simulink model "Tutorial3_part2"  (R2020b)
settings: Solver=FixedStepAuto  StartTime=0.0  StopTime=inf  RelTol=1e-3  EnableMultiTasking=on
settings Model: SILPILModeSetting=veronly  EnablePacing=on  ExtModeTrigDuration=2  Creator=helve  LastModifiedBy=helve
settings OptimizationCC: EnhancedBackFolding=on  PassReuseOutputArgsAs=Individual arguments  ZeroExternalMemoryAtStartup=off  ZeroInternalMemoryAtStartup=off  MaxStackSize=64  OptimizeBlockOrder=speed  DifferentSizesBufferReuse=on  OptimizationCustomize=off  EfficientTunableParamExpr=on
settings DebuggingCC: ParameterTunabilityLossMsg=error
settings HardwareCC: ProdBitPerPointer=32  ProdBitPerSizeT=32  ProdBitPerPtrDiffT=32  ProdLargestAtomicInteger=Long  ProdLargestAtomicFloat=Double  ProdWordSize=32  ProdHWDeviceType=ARM Compatible->ARM Cortex
settings SFSimCC: MATLABDynamicMemAlloc=off
settings RTWCC: Description=Embedded Coder  SystemTargetFile=ert.tlc  HardwareBoard=Arduino Nano 33 IoT  TemplateMakefile=ert_default_tmf  Toolchain=Arduino ARM  BuildConfiguration=Faster Runs
settings CodeAppCC: ForceParamTrailComments=on  IgnoreCustomStorageClasses=off  OperatorAnnotations=on  SimulinkDataObjDesc=on  SFDataObjDesc=on  InsertBlockDesc=on
settings ERTTargetCC: SupportContinuousTime=on  SupportVariableSizeSignals=on  ExtModeStaticAllocSize=8192

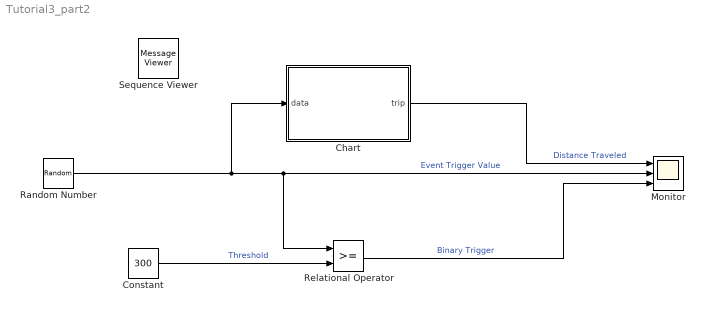
== system Tutorial3_part2 ==
  Chart : Stateflow chart  TreatAsAtomicUnit=on
  Constant : Constant  Value=300
  Monitor : Scope  NumInputPorts=3
  Random Number : RandomNumber  Mean=280  Variance=150  SampleTime=0.1
  Relational Operator : RelationalOperator  OutDataTypeStr=boolean  RndMeth=Simplest
  Sequence Viewer : MessageViewer  History=1000  SavedRootId=#
  wires:
  Random Number/1 -> Relational Operator/1, Monitor/2, Chart/1(data)  "Event Trigger Value"
  Chart/1(trip) -> Monitor/1  "Distance Traveled"
  Constant/1 -> Relational Operator/2  "Threshold"
  Relational Operator/1 -> Monitor/3  "Binary Trigger"

== stateflow chart Tutorial3_part2/Chart ==
  state Driver [parallel]
    settings: executionOrder=1
    state Waiting_In_Parking
      ex:
      trip=data
    state Driving
      du:
      trip=trip-x
    state Reaching_Destination
      en:
      send(DestinationReached,Car)
    (default) -> Waiting_In_Parking
    Waiting_In_Parking -> Driving : [data>300]{send(SthHappened,Car)}
    Driving -> Driving [commented out] : after(1,sec)
    Reaching_Destination -> Waiting_In_Parking : [x==0]
    Driving -> Reaching_Destination : [trip<=0]
  state Car [parallel]
    settings: executionOrder=2
    state Idling
      en:
      x=0;
    state Acceleration
      en:
      x=x+1
    state Decceleration
      en:
      x=x-1
    note: These after transitions can be removed if x is increased based on the step size
    state Cruising
    (default) -> Idling
    Idling -> Acceleration : SthHappened
    (junction 25) -> Idling [order 1] : [x<=0]
    (junction 19) -> Acceleration [order 2]
    Acceleration -> (junction 19) : after(1,sec)
    (junction 25) -> Decceleration [order 2]
    Decceleration -> (junction 25) : after(1,sec)
    Cruising -> Decceleration : DestinationReached
    (junction 19) -> Cruising [order 1] : [x>=10]
  data: data input; x local; trip output
  events: DestinationReached local FUNCTION_CALL_EVENT; SthHappened local FUNCTION_CALL_EVENT
